simulink model "chap17_5sim"  (Simulink 7.7)
settings: Solver=ode45  SolverMode=SingleTasking  StartTime=0.0  StopTime=3  FixedStep=0.001  RelTol=1e-5  AbsTol=1e-5
settings Model: Creator=ljk  LastModifiedBy=ljk  ExtModeTrigMode=oneshot  ExtModeArmWhenConnect=off
settings DataIOCC: LimitDataPoints=off  SignalLoggingName=sigsOut
settings OptimizationCC: BooleanDataType=off  InitFltsAndDblsToZero=on
settings DebuggingCC: SaveWithParameterizedLinksMsg=none  SignalResolutionControl=TryResolveAllWithWarning  SolverPrmCheckMsg=none  MultiTaskDSMMsg=warning  MultiTaskCondExecSysMsg=none  StrictBusMsg=None
settings HardwareCC: TargetUnknown=on
settings RTWCC: IncludeERTFirstTime=on
settings GRTTargetCC: TargetFcnLib=ansi_tfl_tmw.mat

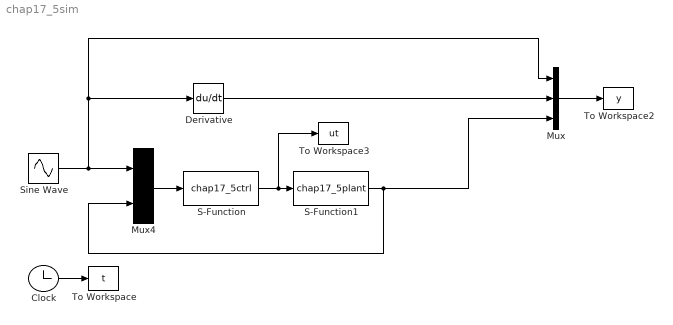
== system chap17_5sim ==
  Clock : Clock
  Derivative : Derivative
  Mux : Mux  Inputs=3
  Mux4 : Mux  Inputs=2
  S-Function : S-Function  FunctionName=chap17_5ctrl  EnableBusSupport=off
  S-Function1 : S-Function  FunctionName=chap17_5plant  EnableBusSupport=off
  Sine Wave : Sin  Amplitude=0.1  Frequency=pi  SampleTime=0
  To Workspace : ToWorkspace  VariableName=t  SampleTime=-1  SaveFormat=Array
  To Workspace2 : ToWorkspace  VariableName=y  SampleTime=-1  SaveFormat=Array
  To Workspace3 : ToWorkspace  VariableName=ut  SampleTime=-1  SaveFormat=Array
  wires:
  Mux4/1 -> S-Function/1
  Mux/1 -> To Workspace2/1
  S-Function/1 -> S-Function1/1, To Workspace3/1
  S-Function1/1 -> Mux4/2, Mux/3
  Sine Wave/1 -> Mux4/1, Mux/1, Derivative/1
  Clock/1 -> To Workspace/1
  Derivative/1 -> Mux/2
